simulink model "Environment_TRC"  (R2013a)
settings: Solver=ode45  StartTime=0.0  StopTime=10.0  RelTol=1e-3
model workspace (MATLAB code in the model file):
  | switch(Env)
  |    case 'Pikes Peak'
  |       load Evn_Pikes_Peak;
  |    case 'IOM'
  |       load Evn_IOM;
  |    otherwise
  |       load Environment
  | end
values from neighbouring files (symbols this model uses):
  altx = [0 1463 2011.6 3216.6 3765.2]    [Environment_TRC.mat]    (also in TRC_testing.m = d)
  alty = [0 0 -5.74 -5.74 0]    [Environment_TRC.mat]    (also in TRC_testing.m = [0,0,-5.74,-5.74,0])
  g = 9.80665    [Environment_TRC.mat]
  L = 0.0065    [Environment_TRC.mat]
  M = 28.9644    [Environment_TRC.mat]
  P0 = 100000    [Environment_TRC.mat]
  R = 8.31432    [Environment_TRC.mat]
  Rcx = [0 1463 2011.6 3216.6 3765.2]    [Environment_TRC.mat]
  Rcy = [233 233 100000 192 10000]    [Environment_TRC.mat]
  T0 = 274    [Environment_TRC.mat]
settings Model: Creator=Nathan  LastModifiedBy=Nathan

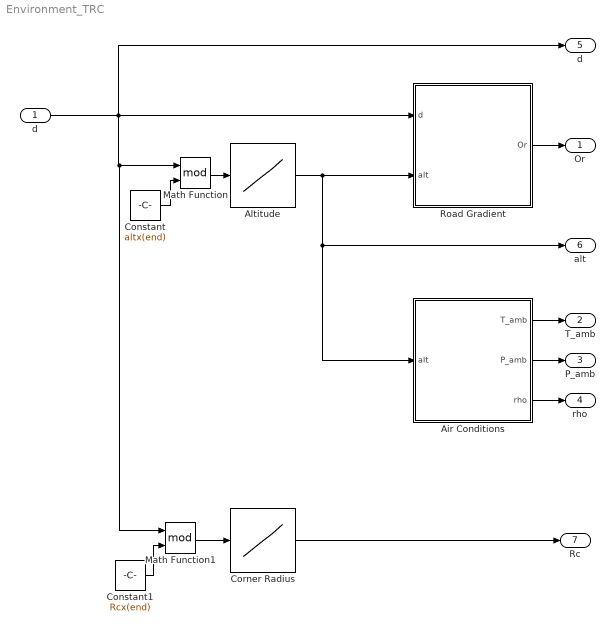
== system Environment_TRC ==
  d : Inport
  Air Conditions : Subsystem
  Altitude : Lookup_n-D  NumberOfTableDimensions=1  BreakpointsForDimension1=altx  Table=alty  ExtrapMethod=Clip  DiagnosticForOutOfRangeInput=Warning  UseLastTableValue=on  RndMeth=Simplest  InputSameDT=on
  Constant : Constant  Value=altx(end)
  Constant1 : Constant  Value=Rcx(end)
  Corner Radius : Lookup_n-D  NumberOfTableDimensions=1  BreakpointsForDimension1=Rcx  Table=Rcy  InterpMethod=Flat  ExtrapMethod=Clip  DiagnosticForOutOfRangeInput=Warning  UseLastTableValue=on  RndMeth=Simplest  InputSameDT=on
  Math Function : Math  Operator=mod  SaturateOnIntegerOverflow=on
  Math Function1 : Math  Operator=mod  SaturateOnIntegerOverflow=on
  Road Gradient : Subsystem
  Or : Outport
  T_amb : Outport  Port=2
  P_amb : Outport  Port=3
  rho : Outport  Port=4
  "d " : Outport  Port=5
  alt : Outport  Port=6
  Rc : Outport  Port=7
  wires:
  Road Gradient/1(Or) -> Or/1
  Altitude/1 -> alt/1, Air Conditions/1(alt), Road Gradient/2(alt)
  Air Conditions/1("T_amb ") -> T_amb/1
  Air Conditions/2(P_amb) -> P_amb/1
  Air Conditions/3(rho) -> rho/1
  Corner Radius/1 -> Rc/1
  d/1 -> Road Gradient/1(d), "d "/1, Math Function1/1, Math Function/1
  Math Function/1 -> Altitude/1
  Math Function1/1 -> Corner Radius/1
  Constant/1 -> Math Function/2
  Constant1/1 -> Math Function1/2

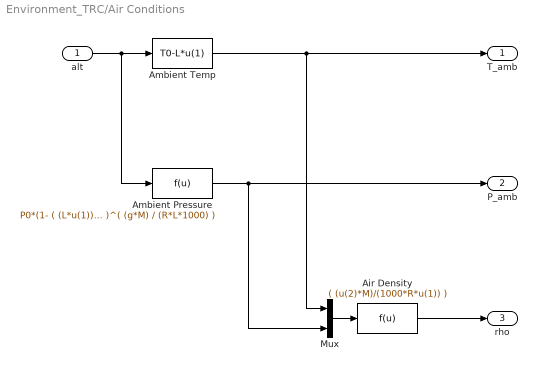
== system Environment_TRC/Air Conditions ==
  alt : Inport
  Air Density : Fcn  Expr=( (u(2)*M)/(1000*R*u(1)) )
  Ambient Pressure : Fcn  Expr=P0*(1- ( (L*u(1))/(T0) ) )^( (g*M) / (R*L*1000) )
  Ambient Temp : Fcn  Expr=T0-L*u(1)
  Mux : Mux  Inputs=2
  "T_amb " : Outport
  P_amb : Outport  Port=2
  rho : Outport  Port=3
  wires:
  alt/1 -> Ambient Pressure/1, Ambient Temp/1
  Ambient Temp/1 -> Mux/1, "T_amb "/1
  Ambient Pressure/1 -> Mux/2, P_amb/1
  Mux/1 -> Air Density/1
  Air Density/1 -> rho/1

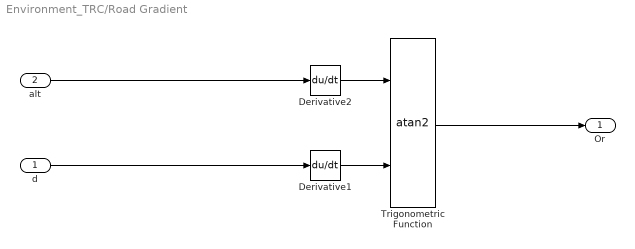
== system Environment_TRC/Road Gradient ==
  d : Inport
  alt : Inport  Port=2
  Derivative1 : Derivative
  Derivative2 : Derivative
  Trigonometric Function : Trigonometry  Operator=atan2
  Or : Outport
  wires:
  alt/1 -> Derivative2/1
  Trigonometric Function/1 -> Or/1
  Derivative1/1 -> Trigonometric Function/2
  d/1 -> Derivative1/1
  Derivative2/1 -> Trigonometric Function/1
